simulink model "diegersh_se_seira"  (R2022a)
settings: Solver=ode23tb  StartTime=0.0  StopTime=3  MaxStep=1e-5  RelTol=1e-3
libraries: spsSeriesRLCBranchLib x9, simulink x4, spsCurrentMeasurementLib x3, spsDCMachineLib x2, spsDCVoltageSourceLib x2, spsControlledCurrentSourceLib x2, spsVoltageMeasurementLib x2, spsControlledVoltageSourceLib x1, spspowerguiLib x1
settings Model: Creator=User  LastModifiedBy=User

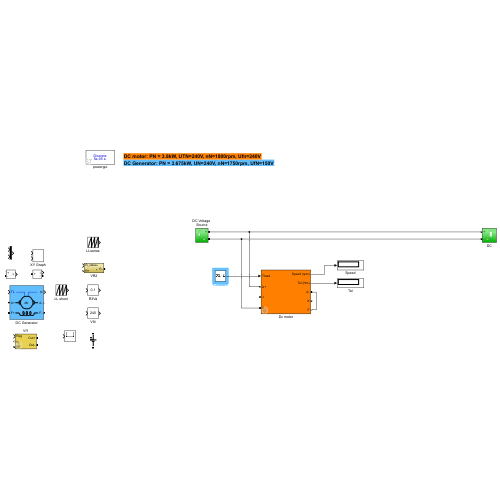
[thumbnail: Simulink's stored preview of the top-level diagram]
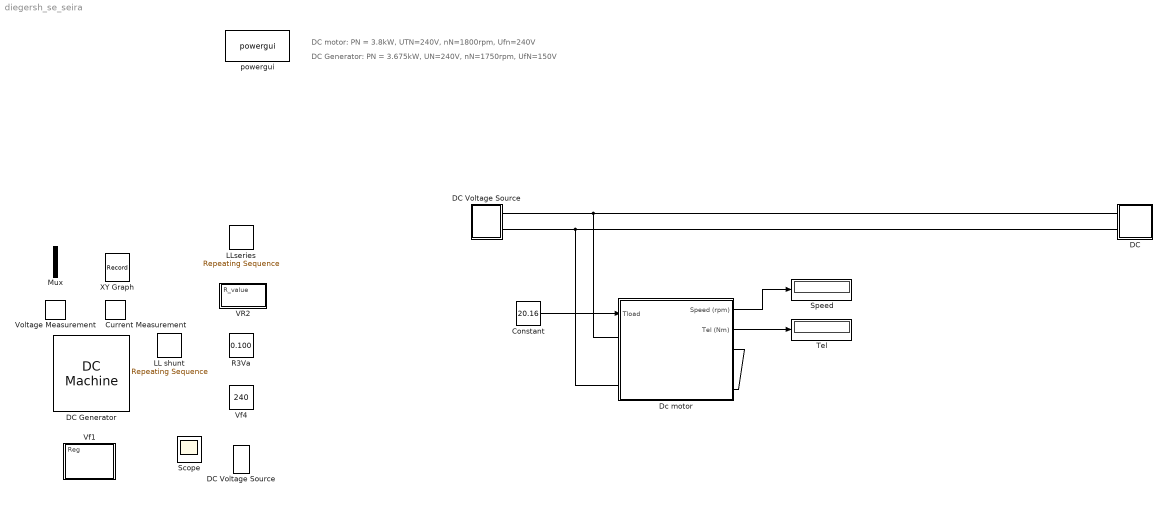
== system diegersh_se_seira ==
  note: DC motor: PN = 3.8kW, UTN=240V, nN=1800rpm, Ufn=240V
  note: DC Generator: PN = 3.675kW, UN=240V, nN=1750rpm, UfN=150V
  Constant : Constant  Value=20.16
  Current Measurement : spsCurrentMeasurementLib/Current Measurement  PhasorSimulation=off  OutputType=Complex  PSBequivalent=0
  DC : Subsystem
  DC Generator : spsDCMachineLib/DC Machine  PresetModel=02: 5HP 240V 1750RPM Field:150V  MechanicalLoad=Torque TL  FieldType=Wound  ShowDetailedParameters=on  MeasurementBus=off  RLa=[0.78 0.016]  RLf=[150 112.5]  Laf=1.234  MachineConstant=Torque constant (N.m/A)  Ke=1.8  Kt=1.8  J=0.05  Bm=0.01  Tf=0  w0=1  Ifinit=0  TsPowergui=0  TsBlock=-1
  DC Voltage Source : Subsystem
  DC Voltage Source : spsDCVoltageSourceLib/DC Voltage Source  Amplitude=0  Measurements=None
  Dc motor : Subsystem  mask{PN=3.8, VN=240, nN=1800}
      mask prompts: PN "PN (kW)"; VN "VN (V)"; nN "nN (rpm)"
      mask DialogControl Control2 Prompt: DC Motor
  LL shunt : simulink/Sources/Repeating Sequence  rep_seq_t=[0 1 2 3 4 5 6 7 8 9 10 11]  rep_seq_y=[0 1.83 3.67 5.5 7.33 9.16 10.97 12.83 14.66 16.49 18.33 20.16]
  LLseries : simulink/Sources/Repeating Sequence  rep_seq_t=[0 1 2 3 4 5 6 7 8 9 10 11]  rep_seq_y=[0 1.83 3.67 5.5 7.33 9.16 10.97 12.83 14.66 16.49 18.33 20.16]
  Mux : Mux  Inputs=2
  R3Va : simulink/Math Operations/Slider Gain  gain=0.100  low=0.1  high=100
  Scope : Scope
  Speed : Display
  Tel : Display
  VR2 : Subsystem
  Vf1 : Subsystem  mask{R=230}
      mask prompts: R "R (Ω)"
      mask DialogControl Label1 Prompt: Variable Resistor
  Vf4 : simulink/Math Operations/Slider Gain  gain=240  low=0  high=240
  Voltage Measurement : spsVoltageMeasurementLib/Voltage Measurement  PhasorSimulation=off  OutputType=Complex  PSBequivalent=0
  XY Graph : Record  FileSettingsInternal="{\"entries\":[{\"content\":{\"excelSettings\":{\"content\":{},\"type\":\"Streamout.ExcelSettings\"}},\"type\":\"Streamout.FileSettingStorage\",\"uuid\":\"4441c915-cd38-4970-a954-959f58e1bd6f\"}],\"packageUris\":[\"http://schema.mathworks.com/mf0/streamout_blocks/R2020a\"],\"version\":\"1.0\"}"  Layout=[1 1]  SignalsInternal="{\"entries\":[{\"content\":{\"signals\":[{\"content\":{\"blockPath\":[\"diegersh_se_seira/XY Graph\"],\"channel\":[],\"dimensions\":[1],\"domain\":\"diegersh_se_seira/XY Graph\",\"lineColor\":\"#a2142f\",\"plots\":[],\"port\":1,\"sid\":[\"\"],\"signalID\":59},\"type\":\"RecordBlkView.Signal\",\"uuid\":\"31a19a27-8fc7-40b7-9868-9ae369d3bc10\"},{\"content\":{\"blockPath\":[\"diegersh_se_seira/XY Graph\"],\"channel\":[],\"dimensions\":[1],\"domain\":\"diegersh_se_seira/XY Graph\",\"lineColor\":\"#139fff\",\"plots\":[],\"port\":2,\"sid\":[\"\"],\"signalID\":63},\"type\":\"RecordBlkView.Signal\",\"uuid\":\"fa413b58-4080-4ab8-ac9e-5a31446b61fa\"}]},\"type\":\"RecordBlkView.InputSignals\",\"uuid\":\"53d354f0-cd89-46a6-8005-a4943c136710\"}],\"packageUris\":[\"http://schema.mathworks.com/mf0/streamout_blocks/R2020a\"],\"version\":\"1.0\"}"  CompatibilityTag=XY  st=-1
  powergui : spspowerguiLib/powergui  Priority=1  SimulationMode=Discrete  SampleTime=50e-6  frequency=60  Iterations=50  frequencyindice=0  Pbase=100e6  ErrMax=1e-4  UnitsV=kV  UnitsW=MW  buscounter=0  FunctionMessages=off  echomessages=off  EnableUseOfTLC=off  CurrentSourceSwitches=off  DisableSnubberDevices=off  DisableRonSwitches=off  DisableVfSwitches=off  DisplayEquations=off  AutomaticDiscreteSolvers=on  SolverType=Tustin/Backward Euler (TBE)  Interpol=off  ExternalGateDelay=off  methode=off  Ts=100  x0status=blocks  SPID=on  SwTol=0  HookPort=off  NonlinearTolerance=1e-4  nMaxIteration=100  ContinueOnMaxIteration=off  RestoreLinks=warning  ResistiveCurrentMeasurement=off  Frange=[0:2:500]  Ylog=off  Xlog=on  ShowGrid=off  save=off  variable=ZData  structure=0  ZoomFFT=off  StartTime=0.0  cycles=1  DisplayStyle=1  fundamental=60  FreqAxis=off  MaxFrequency=1000  frequencyindicesteady=1  RmsSteady=1  display=off
  wires:
  Constant/1 -> Dc motor/1(Tload)
  Dc motor/1(Speed (rpm)) -> Speed/1
  Dc motor/2(Tel (Nm)) -> Tel/1
  connections:
  DC Voltage Source/RConn1 -- Dc motor/LConn1 -- DC/LConn1
  DC Voltage Source/RConn2 -- Dc motor/LConn3 -- DC/LConn2
  Dc motor/RConn1 -- Dc motor/RConn3

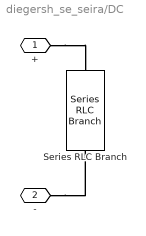
== system diegersh_se_seira/DC ==
  Series RLC Branch : spsSeriesRLCBranchLib/Series RLC Branch  LConnTagsString=__new0  RConnTagsString=__new0  BranchType=R  Resistance=1e4  Inductance=1e-3  SetiL0=off  InitialCurrent=0  Capacitance=1e-6  Setx0=off  InitialVoltage=0  Measurements=None
  + : PMIOPort  Side=Left
  - : PMIOPort  Port=2  Side=Left
  connections:
  -/RConn1 -- Series RLC Branch/RConn1
  +/RConn1 -- Series RLC Branch/LConn1

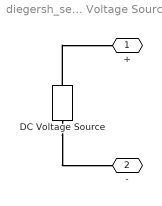
== system diegersh_se_seira/DC Voltage Source ==
  DC Voltage Source : spsDCVoltageSourceLib/DC Voltage Source  Amplitude=240  Measurements=None
  + : PMIOPort  Side=Right
  - : PMIOPort  Port=2  Side=Right
  connections:
  DC Voltage Source/LConn1 -- -/RConn1
  DC Voltage Source/RConn1 -- +/RConn1

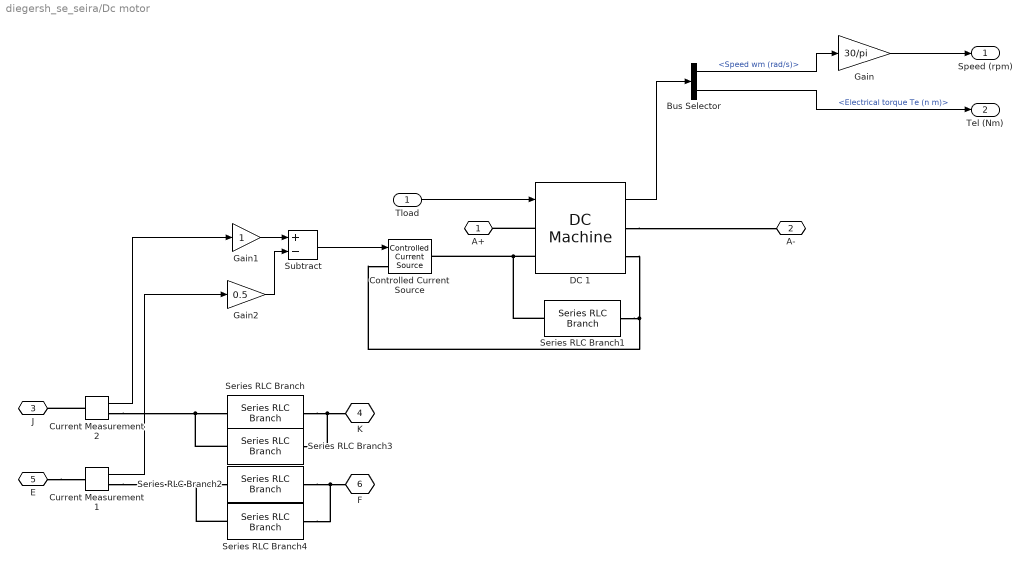
== system diegersh_se_seira/Dc motor ==
  Tload : Inport
  Bus Selector : BusSelector  OutputSignals=Speed wm (rad/s),Electrical torque Te (n m)
  Controlled Current Source : spsControlledCurrentSourceLib/Controlled Current Source  Initialize=on  Source_Type=DC  Amplitude=0  Phase=0  Frequency=0  Measurements=None
  Current Measurement1 : spsCurrentMeasurementLib/Current Measurement  PhasorSimulation=off  OutputType=Complex  PSBequivalent=0
  Current Measurement2 : spsCurrentMeasurementLib/Current Measurement  PhasorSimulation=off  OutputType=Complex  PSBequivalent=0
  DC 1 : spsDCMachineLib/DC Machine  PresetModel=No  MechanicalLoad=Torque TL  FieldType=Wound  ShowDetailedParameters=on  MeasurementBus=off  RLa=[0.78 0.016]  RLf=[150 60]  Laf=1.234  MachineConstant=Torque constant (N.m/A)  Ke=1.8  Kt=1.8  J=0.02  Bm=0.01  Tf=0  w0=0  Ifinit=0  TsPowergui=0  TsBlock=-1
  Gain : Gain  Gain=30/pi
  Gain1 : Gain
  Gain2 : Gain  Gain=0.5
  Series RLC Branch : spsSeriesRLCBranchLib/Series RLC Branch  LConnTagsString=__new0  RConnTagsString=__new0  BranchType=RL  Resistance=240  Inductance=120  SetiL0=off  InitialCurrent=0  Capacitance=1e-6  Setx0=off  InitialVoltage=0  Measurements=None
  Series RLC Branch1 : spsSeriesRLCBranchLib/Series RLC Branch  LConnTagsString=__new0  RConnTagsString=__new0  BranchType=R  Resistance=1e6  Inductance=120  SetiL0=off  InitialCurrent=0  Capacitance=1e-6  Setx0=off  InitialVoltage=0  Measurements=None
  Series RLC Branch2 : spsSeriesRLCBranchLib/Series RLC Branch  LConnTagsString=__new0  RConnTagsString=__new0  BranchType=RL  Resistance=0.1  Inductance=1e-3  SetiL0=off  InitialCurrent=0  Capacitance=1e-6  Setx0=off  InitialVoltage=0  Measurements=None
  Series RLC Branch3 : spsSeriesRLCBranchLib/Series RLC Branch  LConnTagsString=__new0  RConnTagsString=__new0  BranchType=R  Resistance=1e6  Inductance=120  SetiL0=off  InitialCurrent=0  Capacitance=1e-6  Setx0=off  InitialVoltage=0  Measurements=None
  Series RLC Branch4 : spsSeriesRLCBranchLib/Series RLC Branch  LConnTagsString=__new0  RConnTagsString=__new0  BranchType=R  Resistance=1e6  Inductance=120  SetiL0=off  InitialCurrent=0  Capacitance=1e-6  Setx0=off  InitialVoltage=0  Measurements=None
  Subtract : Sum  Inputs=+-
  A+ : PMIOPort  Side=Left
  A- : PMIOPort  Port=2  Side=Right
  J : PMIOPort  Port=3  Side=Left
  K : PMIOPort  Port=4  Side=Right
  E : PMIOPort  Port=5  Side=Left
  F : PMIOPort  Port=6  Side=Right
  Speed (rpm) : Outport
  Tel (Nm) : Outport  Port=2
  wires:
  Current Measurement2/1 -> Gain1/1
  Tload/1 -> DC 1/1
  Gain2/1 -> Subtract/2
  Current Measurement1/1 -> Gain2/1
  Subtract/1 -> Controlled Current Source/1
  Gain1/1 -> Subtract/1
  Bus Selector/2 -> Tel (Nm)/1  "<Electrical torque Te (n m)>"
  Gain/1 -> Speed (rpm)/1
  Bus Selector/1 -> Gain/1  "<Speed wm (rad/s)>"
  DC 1/1 -> Bus Selector/1
  connections:
  Series RLC Branch1/RConn1 -- DC 1/RConn2 -- Controlled Current Source/LConn1
  Series RLC Branch1/LConn1 -- DC 1/LConn2 -- Controlled Current Source/RConn1
  Current Measurement2/RConn1 -- Series RLC Branch3/LConn1 -- Series RLC Branch/LConn1
  DC 1/LConn1 -- A+/RConn1
  Current Measurement2/LConn1 -- J/RConn1
  DC 1/RConn1 -- A-/RConn1
  Series RLC Branch/RConn1 -- Series RLC Branch3/RConn1 -- K/RConn1
  E/RConn1 -- Current Measurement1/LConn1
  Current Measurement1/RConn1 -- Series RLC Branch4/LConn1 -- Series RLC Branch2/LConn1
  Series RLC Branch2/RConn1 -- Series RLC Branch4/RConn1 -- F/RConn1

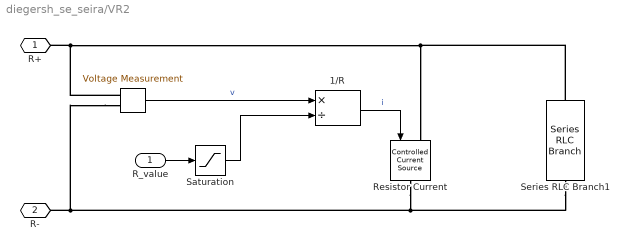
== system diegersh_se_seira/VR2 ==
  R_value : Inport
  " " : spsVoltageMeasurementLib/Voltage Measurement  PhasorSimulation=off  OutputType=Magnitude  PSBequivalent=0
  1/R : Product  Inputs=*/  SaturateOnIntegerOverflow=on  OutDataTypeStr=Inherit: Same as first input
  Resistor Current : spsControlledCurrentSourceLib/Controlled Current Source  Initialize=off  Source_Type=DC  Amplitude=0  Phase=0  Frequency=0  Measurements=None
  Saturation : Saturate  UpperLimit=1e12  LowerLimit=0.01
  Series RLC Branch1 : spsSeriesRLCBranchLib/Series RLC Branch  LConnTagsString=__new0  RConnTagsString=__new0  BranchType=R  Resistance=1e6  Inductance=1e-3  SetiL0=off  InitialCurrent=0  Capacitance=1e-6  Setx0=off  InitialVoltage=0  Measurements=None
  R+ : PMIOPort  Side=Left
  R- : PMIOPort  Port=2  Side=Right
  wires:
  " "/1 -> 1/R/1  "v"
  1/R/1 -> Resistor Current/1  "i"
  R_value/1 -> Saturation/1
  Saturation/1 -> 1/R/2
  connections:
  " "/LConn1 -- Resistor Current/LConn1 -- Series RLC Branch1/LConn1 -- R+/RConn1
  " "/LConn2 -- Series RLC Branch1/RConn1 -- Resistor Current/RConn1 -- R-/RConn1

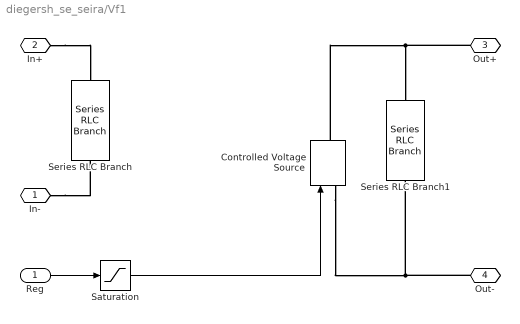
== system diegersh_se_seira/Vf1 ==
  Reg : Inport
  Controlled Voltage Source : spsControlledVoltageSourceLib/Controlled Voltage Source  Initialize=on  Source_Type=DC  Amplitude=0  Phase=0  Frequency=0  Measurements=None
  Saturation : Saturate  UpperLimit=240  LowerLimit=0
  Series RLC Branch : spsSeriesRLCBranchLib/Series RLC Branch  LConnTagsString=__new0  RConnTagsString=__new0  BranchType=R  Resistance=1e6  Inductance=1e-3  SetiL0=off  InitialCurrent=0  Capacitance=1e-6  Setx0=off  InitialVoltage=0  Measurements=None
  Series RLC Branch1 : spsSeriesRLCBranchLib/Series RLC Branch  LConnTagsString=__new0  RConnTagsString=__new0  BranchType=R  Resistance=1e6  Inductance=1e-3  SetiL0=off  InitialCurrent=0  Capacitance=1e-6  Setx0=off  InitialVoltage=0  Measurements=None
  In- : PMIOPort  Side=Left
  In+ : PMIOPort  Port=2  Side=Left
  " Out+" : PMIOPort  Port=3  Side=Right
  " Out-" : PMIOPort  Port=4  Side=Right
  wires:
  Reg/1 -> Saturation/1
  Saturation/1 -> Controlled Voltage Source/1
  connections:
  In+/RConn1 -- Series RLC Branch/LConn1
  In-/RConn1 -- Series RLC Branch/RConn1
  " Out+"/RConn1 -- Controlled Voltage Source/RConn1 -- Series RLC Branch1/LConn1
  " Out-"/RConn1 -- Controlled Voltage Source/LConn1 -- Series RLC Branch1/RConn1
